simulink model "haha"  (R2024b)
settings: Solver=FixedStepAuto  StartTime=0  StopTime=30  FixedStep=0.001  RelTol=1e-3
model workspace (MAT data in the model file):
  x0 = 0
libraries: slpidlib x1
settings Model: Creator=hw  LastModifiedBy=lenovo
settings RTWCC: GPUComputeCapability=3.5

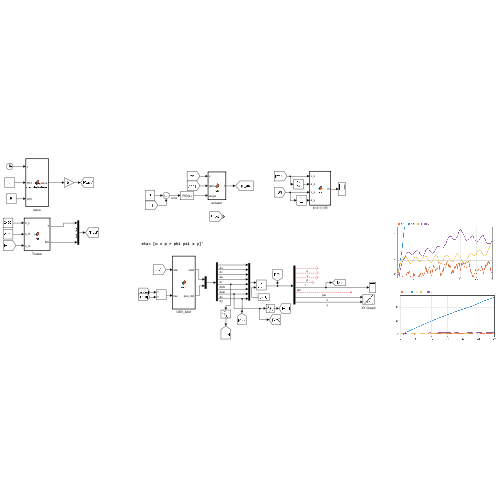
[thumbnail: Simulink's stored preview of the top-level diagram]
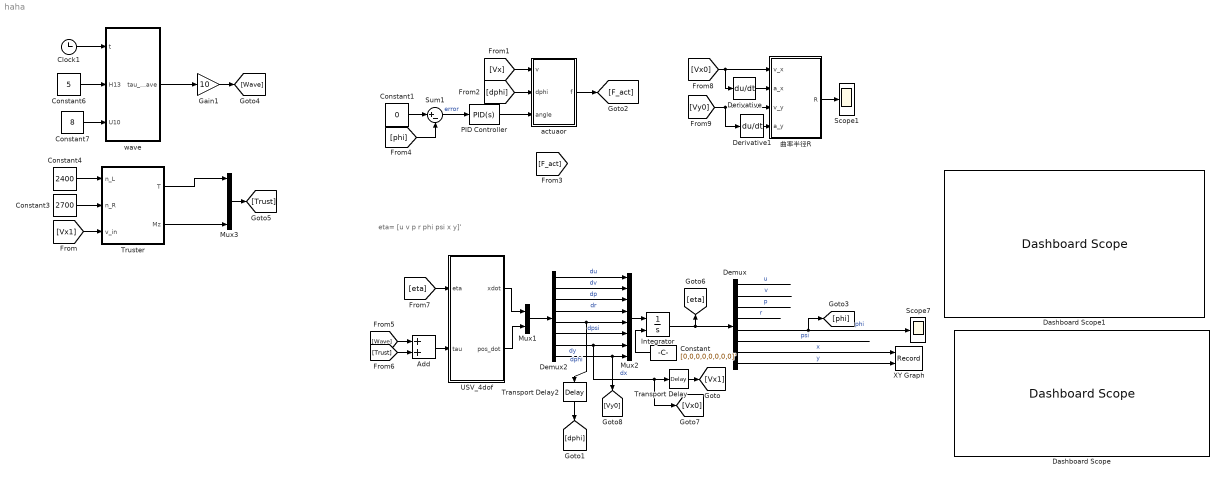
== system haha ==
  note: eta= [u v p r phi psi x y]'
  Add : Sum
  Clock1 : Clock
  Constant : Constant  Value=[0,0,0,0,0,0,0,0]'  VectorParams1D=off
  Constant1 : Constant  Value=0
  Constant3 : Constant  Value=2700
  Constant4 : Constant  Value=2400
  Constant6 : Constant  Value=5
  Constant7 : Constant  Value=8
  Dashboard Scope : DashboardScope
  Dashboard Scope1 : DashboardScope  Ymin=-50  Ymax=50
  Demux : Demux  Outputs=8
  Demux2 : Demux  Outputs=8
  Derivative : Derivative
  Derivative1 : Derivative
  Gain1 : Gain  Gain=10
  Integrator : Integrator  InitialConditionSource=external
  Mux1 : Mux  Inputs=2
  Mux2 : Mux  Inputs=8
  Mux3 : Mux
  PID Controller : slpidlib/PID Controller  Controller=PID  Form=Parallel  TimeDomain=Continuous-time  UseExternalTs=off  SampleTime=-1  IntegratorMethod=Forward Euler  FilterMethod=Forward Euler  ControllerParametersSource=internal  P=6  I=0.7  UseKiTs=off  D=3  UseExternalDerivativeSource=off  N=100  UseFilter=on  TunerSelectOption=Transfer Function Based (PID Tuner App)  InitialConditionSource=internal  InitialConditionForIntegrator=0  InitialConditionForFilter=0  DifferentiatorICPrevScaledInput=0  ExternalReset=none  TrackingMode=off  Kt=1  LimitOutput=off  SatLimitsSource=internal  UpperSaturationLimit=inf  LowerSaturationLimit=-inf  LinearizeAsGain=on  AntiWindupMode=none  Kb=1  LimitIntegrator=off  UpperIntegratorSaturationLimit=inf  LowerIntegratorSaturationLimit=-inf  POutMin=[]  POutMax=[]  IOutMin=[]  IOutMax=[]  DOutMin=[]  DOutMax=[]  NOutMin=[]  NOutMax=[]  SumOutMin=[-15]  SumOutMax=[15]  SaturationOutMin=[]  SaturationOutMax=[]  PParamMin=[]  PParamMax=[]  IParamMin=[]  IParamMax=[]  DParamMin=[]  DParamMax=[]  NParamMin=[]  NParamMax=[]  KbParamMin=[]  KbParamMax=[]  KtParamMin=[]  KtParamMax=[]  KbOutMin=[]  KbOutMax=[]  KtOutMin=[]  KtOutMax=[]  IntegratorOutMin=[]  IntegratorOutMax=[]  FilterOutMin=[]  FilterOutMax=[]  SumI1OutMin=[]  SumI1OutMax=[]  SumI2OutMin=[]  SumI2OutMax=[]  SumI3OutMin=[]  SumI3OutMax=[]  SumI4OutMin=[]  SumI4OutMax=[]  SumDOutMin=[]  SumDOutMax=[]  DifferentiatorOutMin=[]  DifferentiatorOutMax=[]  FilterDiffOutCoefMin=[]  FilterDiffOutCoefMax=[]  ReciprocalOutMin=[]  ReciprocalOutMax=[]  SumDenOutMin=[]  SumDenOutMax=[]  SumNumOutMin=[]  SumNumOutMax=[]  DivideOutMin=[]  DivideOutMax=[]  UdiffTsProdOutMin=[]  UdiffTsProdOutMax=[]  NTsProdOutMin=[]  NTsProdOutMax=[]  UintegralTsProdOutMin=[]  UintegralTsProdOutMax=[]  UngainTsProdOutMin=[]  UngainTsProdOutMax=[]  ClampingZeroOutDataTypeStr=Inherit: Inherit via back propagation  ClampingZeroOutMin=[]  ClampingZeroOutMax=[]  FilterDenConstantOutDataTypeStr=Inherit: Inherit via back propagation  FilterDenConstantOutMin=[]  FilterDenConstantOutMax=[]  PCopyOutDataTypeStr=Inherit: Inherit via back propagation  PCopyOutMin=[]  PCopyOutMax=[]  NCopyOutDataTypeStr=Inherit: Inherit via back propagation  NCopyOutMin=[]  NCopyOutMax=[]  IntegratorContinuousStateAttributes=''  IntegratorStateMustResolveToSignalObject=off  IntegratorRTWStateStorageClass=Auto  FilterContinuousStateAttributes=''  FilterStateMustResolveToSignalObject=off  FilterRTWStateStorageClass=Auto  ParallelPVariant=InternalParameters  IdealPVariant=Disabled  IVariant=InternalParameters  DVariant=InternalParameters  IntegratorVariant=Continuous  SatVariant=Disabled  AWVariant=Passthrough  PCopyVariant=Disabled  TRVariant=Disabled  FdbkBlocksVariant=Forward  IdealPFdbkVariant=Disabled  SatFdbkVariant=Disabled  DerivativeFilterVariant=ContFilter  NVariant=InternalParameters  NCopyVariant=Disabled  FilterICVariant=InternalICsFilter  IntegratorICVariant=InternalICs  ExternalResetVariant=Disabled  TRSumVariant=Passthrough  SumFdbkVariant=Disabled  SumVariant=Sum_PID  TsampFilterVariant=InternalTs  TsampNgainVariant=Passthrough  TsampIntegralVariant=Disabled_SignalSpec  ExternalSaturationOutDataTypeStr=Inherit: Same as second input  DerivativeSourceVariant=ErrorSignal  PreIntVariant=InternalPreInt
  Scope1 : Scope
  Scope7 : Scope
  Sum1 : Sum  Inputs=|+-
  Transport Delay : TransportDelay  DelayTime=0.3
  Transport Delay2 : TransportDelay  DelayTime=0.25
  Truster : MATLAB Function  TreatAsAtomicUnit=on
  USV_4dof : MATLAB Function  TreatAsAtomicUnit=on
  XY Graph : Record  FileSettingsInternal="{\"entries\":[{\"content\":{\"excelSettings\":{\"content\":{},\"type\":\"Streamout.ExcelSettings\"}},\"type\":\"Streamout.FileSettingStorage\",\"uuid\":\"\"}],\"packageUris\":[\"http:\\/\\/schema.mathworks.com\\/mf0\\/streamout_blocks\\/R2020a\"],\"version\":\"1.0\"}"  Layout=[1 1]  SignalsInternal="{\"entries\":[{\"content\":{\"signals\":[{\"content\":{\"blockPath\":[],\"dimensions\":[1,1],\"domain\":\"\",\"lineColor\":\"#a2142f\",\"plots\":[ 1 ],\"port\":1,\"sid\":[\"\"],\"signalID\":1,\"signalName\":\"x\"},\"type\":\"RecordBlkView.Signal\",\"uuid\":\"\"},{\"content\":{\"blockPath\":[],\"dimensions\":[1,1],\"domain\":\"\",\"lineColor\":\"#139fff\",\"plots\":[ 1 ],\"port\":2,\"sid\":[\"\"],\"signalID\":2,\"signalName\":\"y\"},\"type\":\"RecordBlkView.Signal\",\"uuid\":\"\"}]},\"type\":\"RecordBlkView.InputSignals\",\"uuid\":\"\"}],\"packageUris\":[\"http:\\/\\/schema.mathworks.com\\/mf0\\/streamout_blocks\\/R2020a\"],\"version\":\"1.0\"}"  VisualizationBindings="{\"xyplotplugin\":{\"info\":[{\"series\":[{\"bindingParametersList\":[{\"parameter\":\"X-Axis\",\"signalID\":1,\"signalName\":\"x\"},{\"parameter\":\"Y-Axis\",\"signalID\":2,\"signalName\":\"y\"}],\"seriesID\":0}],\"subplotID\":1}]}}"  CompatibilityTag=XY
  actuaor : MATLAB Function  TreatAsAtomicUnit=on
  wave : MATLAB Function  TreatAsAtomicUnit=on
  曲率半径R : MATLAB Function  TreatAsAtomicUnit=on
  wires:
  USV_4dof/1(xdot) -> Mux1/1
  USV_4dof/2(pos_dot) -> Mux1/2
  Mux1/1 -> Demux2/1
  Integrator/1 -> Demux/1, [eta]
  Demux/7 -> XY Graph/1  "x"
  Demux/8 -> XY Graph/2  "y"
  Demux/6 -> ?  "psi"
  Demux/1 -> ?  "u"
  Demux/2 -> ?  "v"
  Demux/3 -> ?  "p"
  Demux/4 -> ?  "r"
  Constant/1 -> Integrator/2
  Clock1/1 -> wave/1(t)
  Constant6/1 -> wave/2(H13)
  Constant7/1 -> wave/3(U10)
  Demux2/1 -> Mux2/1  "du"
  Demux2/2 -> Mux2/2  "dv"
  Demux2/3 -> Mux2/3  "dp"
  Demux2/4 -> Mux2/4  "dr"
  Demux2/5 -> Mux2/5, Transport Delay2/1  "dphi"
  Demux2/6 -> Mux2/6  "dpsi"
  Demux2/7 -> Mux2/7, [Vx0], Transport Delay/1  "dx"
  Demux2/8 -> Mux2/8, [Vy0]  "dy"
  Mux2/1 -> Integrator/1
  Derivative/1 -> 曲率半径R/2(a_x)
  Derivative1/1 -> 曲率半径R/4(a_y)
  曲率半径R/1(R) -> Scope1/1
  Constant3/1 -> Truster/2(n_R)
  Truster/1(T) -> Mux3/1
  Truster/2(Mz) -> Mux3/4
  Constant4/1 -> Truster/1(n_L)
  Add/1 -> USV_4dof/2(tau)
  Constant1/1 -> Sum1/1
  Sum1/1 -> PID Controller/1  "error"
  wave/1(tau_wave) -> Gain1/1
  Transport Delay/1 -> [Vx1]
  Transport Delay2/1 -> [dphi]
  [dphi] -> actuaor/2(dphi)
  actuaor/1(f) -> [F_act]
  [Vx] -> actuaor/1(v)
  PID Controller/1 -> actuaor/3(angle)
  [phi] -> Sum1/2
  Gain1/1 -> [Wave]
  Mux3/1 -> [Trust]
  [Trust] -> Add/2
  [eta] -> USV_4dof/1(eta)
  [Vx0] -> Derivative/1, 曲率半径R/1(v_x)
  [Vy0] -> Derivative1/1, 曲率半径R/3(v_y)
  Demux/5 -> Scope7/1, [phi]  "phi"
  [Wave] -> Add/1
  [Vx1] -> Truster/3(v_in)

== matlab function haha/USV_4dof ==
  data: eta input size=8*1; xdot output size=6*1; tau input; pos_dot output size=2*1
function [xdot,pos_dot] = usv(eta, tau)

% 线性化船舶模型
% Inputs:
% eta= [u v p r phi psi x y]'
% xdot= [du dv dp dr dphi dpsi]'
% pos_dot=[dx dy]'
% tau = [Xe Ye Ke Ne]' 
%
% where
% u     = surge velocity          (m/s)
% v     = sway velocity           (m/s)
% p     = roll velocity           (rad/s)
% r     = yaw velocity            (rad/s)
% phi   = roll angle              (rad)
% psi   = yaw angle               (rad)
%
% Xe is the surge external force (e.g. rudder and fin forces)
% Ye is the sway external force  
% Ke is the sway external force  
% Ne is the sway external force   

% Vessel Data
rho_water     =	1014.0;	        %	water density	[kg/m^3]	
rho_air		=	1.225	;	    %	air density		[kg/m^3]	
g				=	9.81;	        %	gravity constant	[m/s^2]	
deg2rad 		=	pi/180;	        %	degrees to radians	
rad2deg 		=	180/pi;	        %	rad to degrees		
ms2kt			=	3600/1852;	    % 	m/s to kt 			
kt2ms 		=	1852/3600;	    %	kt to m/s			
RPM2rads		=	2*pi/60;	    %	RPM to rad/s		
rads2RPM		=   60/(2*pi);	    %	rad/s to RPM		
HP2W			=	745.700;	    %	HP to Watt			

Lpp    =  3.5 ;                  % Length between perpendiculars垂直间长 [m]
B      =  3.6  ;                  % Beam over all 船宽 [m]
D	   =  0.4  ;                  % Draught吃水深度 [m]     

%Load condition (Modified by T.Perez)
disp   =  0.357;                   % Displacement 排水量 [m^3]
m      =  disp*rho_water;          % Mass [Kg]
Izz    =  213.55 ;            % Yaw Inertia偏航转动惯量
Ixx    =  48.3 ;            % Roll Inertia横滚转动惯量
U_nom  =  8.0   ;	               % Speed nominal [m/sec]速度 (app 15kts) 
KM		=  1.47;	             %  [m] Transverse metacentre above keel 横倾复原力臂
KB		=  0.53;	             %  [m] Transverse centre of bouancy 浮心高度
gm 		=  0.5;	                 %  [m]	Transverse Metacenter 
bm 		=  KM - KB;
LCG       = 20.41 ;                % [m]	Longitudinal CG (from AP considered at the rudder stock)
VCG       = 1.36  ;                % [m]	Vertical  CG  above baseline
xG        = -1.38  ;               % coordinate of CG from the body fixed frame adopted for the PMM test  
zG  	    = -(VCG-D);          % coordinate of CG from the body fixed frame adopted for the PMM test  
m_xg	    = m * xG;
m_zg	    = m * zG;
Dp        = 1.6 ;                   % Propeller diameter [m]


% Data for surge equation 纵向（均为线性流体动力导数）
Xudot  	= -174.000 ;  %-mx
Xuau     	= -460 ;
Xvr    	=  0.33 * m ;
   
% Hydrodynamic coefficients in sway equation横向
Yvdot = -3930 ;  %-my
Ypdot = -296 ; 
Yrdot = -1400 ; %附加质量静距
Yauv  = -11.8 ; 
Yur   =  131 ; 
Yvav  = -3700 ; 
Yrar   =  0 ;
Yvar  = -794 ; 
Yrav  = -182 ; 
Ybauv =  10.800 ; % Y_{\phi |v u|}
Ybaur =  251.000 ; 
Ybuu  = -0.074 ; 


% Hydrodynamic coefficients in roll equation横摇水动力系数
Kvdot =  196.000 ;
Kpdot = -77.4000 ;  %-Jxx
Krdot =  0 ;
Kauv  =  39.260 ;
Kur   = -102.000 ;
Kvav  =  29.300 ;
Krar  =  0 ;
Kvar  =  621.000 ;
Krav  =  14.2000 ;
Kbauv =  -18.400 ;
Kbaur =  -19.6000 ;
Kbuu  =  -11.80 ;
Kaup  =  -155.00 ;
Kpap  =  -416.000 ;
Kp    =  -50.000 ;
Kb    =  0.176*m*g;
Kbbb  =  -0.005*m*g ;

% Hydrodynamic coefficients in yaw equation偏航水动力系数
Nvdot =  538.000 ;   %-
Npdot =  0 ;
Nrdot = -387;    %jzz
Nauv  = -520.00 ;
Naur  = -1710.000 ;
Nvav  =  0 ;
Nrar  = -202.000000 ;
Nvar  =  0 ;
Nrav  = -156.00000 ;
Nbauv = -214.000 ;
Nbuar = -498.0000 ;
Nbuau = -8.000 ;
%%%%%%%%%%%%%%%%%%%%%%%%%%%%%%%%%%%%%%%%%%%%%%%%%%%%%%%%%%%%%%%%%%%%%%%%%%%

% 定义输入
u   = eta(1);
v   = eta(2);
p  	= eta(3);   	
r  	= eta(4); 
b  	= eta(5); %phi roll 		
psi = eta(6);
x  	= eta(7);   	
y  	= eta(8); 
% 外部力与力矩
Xe  = tau(1);
Ye  = tau(2);
Ke  = tau(3);
Ne  = tau(4);


d=0.5;  %横向距离

% Auxiliary variables辅助变量
au = abs(u);
av = abs(v); 
ar = abs(r); 
ap = abs(p); 
ab = abs(b);
L2 = Lpp^2; %参考面积？

% Total Mass Matrix 刚体质量矩阵
% x= [u v p r phi psi ]'
M =[ (m-Xudot)  0   0   0   0   0;
   0 (m-Yvdot) -(m*zG+Ypdot) (m*xG-Yrdot) 0 0;
   0 -(m*zG+Kvdot) (Ixx-Kpdot) -Krdot 0 0;
   0 (m*xG-Nvdot) -Npdot (Izz-Nrdot) 0 0;
   0 0 0 0 1 0; 
   0 0 0 0 0 1] ;
%转换矩阵
J=[cos(psi),-cos(b)*sin(psi);sin(psi),cos(b)*cos(psi)];
X=[u,v]';   
% Hydrodynamic forces without added mass terms(considered in the M matrix)
% 不考虑附加质量的水动力作用力 粘性流动动力（贵岛模型）
Xh  = Xuau*u*au+Xvr*v*r;

Yh = Yauv*au*v +  Yur*u*r + Yvav*v*av + Yvar*v*ar + Yrav*r*av + Ybauv*b*abs(u*v) + Ybaur*b*abs(u*r) + Ybuu*b*u^2;

Kh = Kauv*au*v +Kur*u*r + Kvav*v*av + Kvar*v*ar + Krav*r*av + Kbauv*b*abs(u*v) + Kbaur*b*abs(u*r) + Kbuu*b*u^2 +Kaup*au*p + Kpap*p*ap +Kp*p +Kbbb*b^3-(rho_water*g*gm*disp)*b;

Nh =Nauv*au*v + Naur*au*r +Nrar*r*ar + Nrav*r*av+Nbauv*b*abs(u*b) + Nbuar*b*u*ar + Nbuau*b*u*au;
 
% Rigid-body centripetal accelerations刚体运动产生的离心加速度影响
Xc =  m*(r*v+xG*r^2-zG*p*r);  
Yc = - m*u*r;
Kc =   m*zG*u*r;
Nc = - m*xG*u*r;

% Total forces
F1 = Xh+Xc+Xe;
F2 = Yh+Yc+Ye;
F4 = Kh+Kc+Ke;
F6 = Nh+Nc+Ne;
%运动学及动力学方程
pos_dot=J*X;
xdot = M\[F1; F2; F4; F6; p; r*cos(b)];

end

== matlab function haha/wave ==
  settings: updateMethod=DISCRETE
  data: t input; tau_wave output; H13 input; U10 input
function tau_wave = wave_disturbance(t, H13, U10)
    % 计算波浪干扰力矩
    % 输入参数：
    % t         - 时间 [s]
    % H13       - 有效波高 [m]
    % U10       - 风速 [m/s]
    % beta      - 船舶与海浪的遭遇角 [rad]
    
    % 常数定义
    g = 9.81;               % 重力加速度, m/s^2
    alpha_pm = 8.11e-3;     % Pierson-Moskowitz谱参数
    beta_pm = 3.11;         % Pierson-Moskowitz谱参数
    beta=pi/4;
    % 计算峰值频率
    omega_peak = 0.84 * (g / U10)^(1/3); % 峰值频率, rad/s
    
    % 根据H13确定频率范围和步长
    if H13 <= 2.5
        omegab = 0.3;
        omegal = 3.0;
        delta_omega = 0.1;
    elseif H13 <= 5.0
        omegab = 0.25;
        omegal = 2.4;
        delta_omega = 0.08;
    else 
        omegab = 0.1;
        omegal = 1.7;
        delta_omega = 0.06;
    end
    omega = omegab:delta_omega:omegal;
    
    % 计算海浪能谱
    S_omega = alpha_pm * g^2 ./ omega.^5 .* exp(-beta_pm ./ (H13^2 * omega.^4));
    
    % 计算各频率成分的振幅和相位
    A = sqrt(2 * S_omega * delta_omega);
    phi = rand(1, length(omega)) * 2 * pi; % 随机相位
    
    % 船舶参数
    rho = 1024; % 海水密度 [kg/m^3]
    L = 3.5;     % 船长 [m]
    B = 1.8;     % 船宽 [m]
    D = 0.4;     % 吃水深度 [m]
    
    % 初始化波浪干扰力矩分量
    tao1 = zeros(size(t));
    tao2 = zeros(size(t));
    tao3 = zeros(size(t)); % 第三分量保持为零
    tao4 = zeros(size(t));
    
    % 计算各频率成分对力矩的贡献
    for i = 1:length(omega)
        k = omega(i)^2 / g;           % 波数（深水条件）
        omega_e = omega(i);           % 遭遇频率（假设船速为零）
        phase = omega_e * t + phi(i); % 相位项
        slope_term = k * A(i) * sin(phase); % 波面斜率相关项
        
        % 纵向力矩
        tao1 = tao1 + rho * g * B * L * D * cos(beta) * slope_term;
        % 横向力矩
        tao2 = tao2 - rho * g * B * L * D * sin(beta) * slope_term;
        % 横摇力矩（假设公式正确性）
        tao4 = tao4 + (1/24) * rho * g * B * L * (L^2 - B^2) * sin(2*beta) * (slope_term)^2;
    end
    
    % 组合力矩分量
    tau_wave = [tao1; tao2;tao2; tao4];
end

== matlab function haha/曲率半径R ==
  data: v_x input; a_x input; R output; v_y input; a_y input
function R   = top(v_x,a_x, v_y,a_y)

R=sqrt((v_x^2+v_y^2)^3)/abs(v_x*a_y-v_y*a_x);
end

== matlab function haha/Truster ==
  data: n_L input; n_R input; T output; v_in input; Mz output
function [T , Mz] = fcn(n_L,n_R,v_in)

%% 常量定义
rho=1024;
%模型泵参数

Q0=0.523;  %换算流量
D0=0.3048;  %叶轮直径
n0=1450;    %转速

%现有泵参数
D=0.14;   %叶轮直径
d=0.098;   %喷嘴直径
d_eff = 1.6;  %喷嘴间距
Q_L=Q0*(n_L/n0)*(D/D0)^3;
Q_R=Q0*(n_R/n0)*(D/D0)^3;
%% 推力换算
v_jL=4*Q_L/(pi*d*d);
v_jR=4*Q_R/(pi*d*d);
T_L=rho*Q_L*(v_jL-v_in);
T_R=rho*Q_R*(v_jR-v_in);
T=T_R+T_L;
Mz=(T_R-T_L)*  d_eff ;

== matlab function haha/actuaor ==
  data: v input; dphi input; angle input size=1*1; f output size=1*1
function f  = top(v, dphi, angle)

d=2;
f=1/2*v^2*1025*10*0.87*(angle+dphi*d);
end
